simulink model "swirling_pendulum_PFL_acrobot_spong_based_collocated"  (R2021a)
settings: Solver=ode2  StartTime=0.0  StopTime=40  FixedStep=1e-4  RelTol=1e-3
undefined symbols (not defined in the file or in its folder): sigbuilder_block, X, Y, Z
libraries: sm_lib x15, nesl_utility x3, dspswit3 x1
settings Model: Creator=aarti  LastModifiedBy=Riswadkar
settings SolverCC: ZeroCrossControl=DisableAll
settings DataIOCC: SaveState=on  ReturnWorkspaceOutputs=off

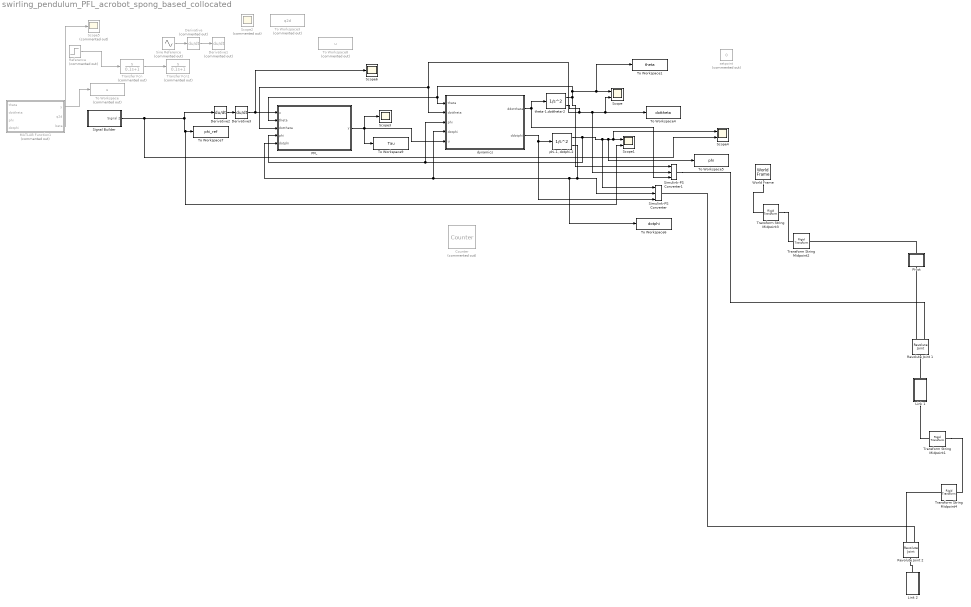
== system swirling_pendulum_PFL_acrobot_spong_based_collocated ==
  Counter : dspswit3/Counter  Commented=on  Direction=Up  CountEvent=Rising edge  CounterSize=User defined  MaxCount=255  InitialCount=0  Output=Count and Hit  HitValue=32  ResetInput=on  SamplesPerFrame=1  Ts=1  CntDtype=double  HitDtype=Logical
  Derivative : Derivative  Commented=on
  Derivative1 : Derivative  Commented=on
  Derivative2 : Derivative
  Derivative3 : Derivative
  Link 1 : Subsystem  Tag=CustomStyle
  Link 2 : Subsystem  Tag=CustomStyle
  MATLAB Function1 : MATLAB Function  Commented=on  TreatAsAtomicUnit=on
  PFL : MATLAB Function  TreatAsAtomicUnit=on
  Pivot : Subsystem  Tag=CustomStyle
  Reference : Step  Commented=on  Time=2  After=pi/2  SampleTime=0
  Revolute Joint 1 : sm_lib/Joints/Revolute Joint  JointMode=Normal  SenseConstraintForce=off  SenseConstraintForceX=off  SenseConstraintForceY=off  SenseConstraintForceZ=off  SenseConstraintTorque=off  SenseConstraintTorqueX=off  SenseConstraintTorqueY=off  SenseConstraintTorqueZ=off  SenseTotalForce=off  SenseTotalForceX=off  SenseTotalForceY=off  SenseTotalForceZ=off  SenseTotalTorque=off  SenseTotalTorqueX=off  SenseTotalTorqueY=off  SenseTotalTorqueZ=off  CompositeWrenchDir=FollowerOnBase  CompositeWrenchFrame=BaseFrame  EquilibriumPosition=0  EquilibriumPositionUnits=rad  SpringStiffness=0  SpringStiffnessUnits=N*m/rad  DampingCoefficient=0  DampingCoefficientUnits=N*m/(rad/s)  TorqueActuationMode=ComputedTorque  MotionActuationMode=InputMotion  SensePosition=off  SenseVelocity=off  SenseAcceleration=off  SenseTorqueForce=off  SenseLowerLimitTorqueForce=off  SenseUpperLimitTorqueForce=off  LowerLimitSpecify=off  LowerLimitBound=-90  LowerLimitBoundUnits=deg  LowerLimitStiffness=1e4  LowerLimitStiffnessUnits=N*m/deg  LowerLimitDamping=10  LowerLimitDampingUnits=N*m/(deg/s)  LowerLimitTransitionRegionWidth=0.1  LowerLimitTransitionRegionWidthUnits=deg  UpperLimitSpecify=off  UpperLimitBound=90  UpperLimitBoundUnits=deg  UpperLimitStiffness=1e4  UpperLimitStiffnessUnits=N*m/deg  UpperLimitDamping=10  UpperLimitDampingUnits=N*m/(deg/s)  UpperLimitTransitionRegionWidth=0.1  UpperLimitTransitionRegionWidthUnits=deg  PositionTargetSpecify=off  PositionTargetPriority=High  PositionTargetValue=0  PositionTargetValueUnits=deg  VelocityTargetSpecify=off  VelocityTargetPriority=High  VelocityTargetValue=0  VelocityTargetValueUnits=rad/s
  Revolute Joint 2 : sm_lib/Joints/Revolute Joint  JointMode=Normal  SenseConstraintForce=off  SenseConstraintForceX=off  SenseConstraintForceY=off  SenseConstraintForceZ=off  SenseConstraintTorque=off  SenseConstraintTorqueX=off  SenseConstraintTorqueY=off  SenseConstraintTorqueZ=off  SenseTotalForce=off  SenseTotalForceX=off  SenseTotalForceY=off  SenseTotalForceZ=off  SenseTotalTorque=off  SenseTotalTorqueX=off  SenseTotalTorqueY=off  SenseTotalTorqueZ=off  CompositeWrenchDir=FollowerOnBase  CompositeWrenchFrame=BaseFrame  EquilibriumPosition=0  EquilibriumPositionUnits=rad  SpringStiffness=0  SpringStiffnessUnits=N*m/rad  DampingCoefficient=0  DampingCoefficientUnits=N*m/(rad/s)  TorqueActuationMode=ComputedTorque  MotionActuationMode=InputMotion  SensePosition=off  SenseVelocity=off  SenseAcceleration=off  SenseTorqueForce=off  SenseLowerLimitTorqueForce=off  SenseUpperLimitTorqueForce=off  LowerLimitSpecify=off  LowerLimitBound=-90  LowerLimitBoundUnits=deg  LowerLimitStiffness=1e4  LowerLimitStiffnessUnits=N*m/deg  LowerLimitDamping=10  LowerLimitDampingUnits=N*m/(deg/s)  LowerLimitTransitionRegionWidth=0.1  LowerLimitTransitionRegionWidthUnits=deg  UpperLimitSpecify=off  UpperLimitBound=90  UpperLimitBoundUnits=deg  UpperLimitStiffness=1e4  UpperLimitStiffnessUnits=N*m/deg  UpperLimitDamping=10  UpperLimitDampingUnits=N*m/(deg/s)  UpperLimitTransitionRegionWidth=0.1  UpperLimitTransitionRegionWidthUnits=deg  PositionTargetSpecify=off  PositionTargetPriority=High  PositionTargetValue=0  PositionTargetValueUnits=deg  VelocityTargetSpecify=off  VelocityTargetPriority=High  VelocityTargetValue=0  VelocityTargetValueUnits=rad/s
  Scope : Scope  NumInputPorts=2
  Scope1 : Scope  NumInputPorts=2
  Scope2 : Scope  Commented=on
  Scope3 : Scope
  Scope4 : Scope  NumInputPorts=2
  Scope5 : Scope  Commented=on
  Scope6 : Scope
  Signal Builder : Subsystem  Tag=STV Subsys  LoadFcn=sigbuilder_block('load');  StartFcn=sigbuilder_block('start');  StopFcn=sigbuilder_block('stop');  ClipboardFcn=sigbuilder_block('clipboard');  mask(Sigbuilder block){tuvar=[0:10]}
      mask help: Simulink:masks:SigbuilderBlock_MD
      mask init:
      | if ~strcmp(get_param(bdroot(gcbh),'SimulationStatus'),'stopped') tuvar = sigbuilder_block('maskInit'); end
      settings: CopyFcn=sigbuilder_block('copy');  DeleteFcn=sigbuilder_block('delete');  ModelCloseFcn=sigbuilder_block('modelClose');  PreSaveFcn=sigbuilder_block('preSave');  PauseFcn=sigbuilder_block('pause');  ContinueFcn=sigbuilder_block('continue');  NameChangeFcn=sigbuilder_block('namechange');  OpenFcn=sigbuilder_block('open',[5.4 36 1141.2 516.6 ]);  CloseFcn=sigbuilder_block('close');
      mask Display: plot(0, 0, 100, 100,[2, 2, 32, 32, 2], [68, 8, 8, 68, 68],[32, 2], [38, 38], [32, 19, 2],[53, 60, 44], [32, 17, 17, 2],[16, 16, 31, 31]);txt = getActiveGroup(gcbh);text(2, 100, txt,'verticalAlignment', 'top');
  Simulink-PS Converter : nesl_utility/Simulink-PS Converter  PhysicalDomain=network_engine_domain  SubClassName=ps_input  LeftPortType=input  RightPortType=output  PseudoPeriodic=off  Frequencies=[]  NoiseDistribution=none  NoiseParameters=[]  Unit=1  AffineConversion=off  FilteringAndDerivatives=provide  SimscapeFilterOrder=1  InputFilterTimeConstant=0.001  UdotUserProvided=2
      settings: SourceProductBaseCode=PW,SS
  Simulink-PS Converter1 : nesl_utility/Simulink-PS Converter  PhysicalDomain=network_engine_domain  SubClassName=ps_input  LeftPortType=input  RightPortType=output  PseudoPeriodic=off  Frequencies=[]  NoiseDistribution=none  NoiseParameters=[]  Unit=1  AffineConversion=off  FilteringAndDerivatives=provide  SimscapeFilterOrder=1  InputFilterTimeConstant=0.001  UdotUserProvided=2
      settings: SourceProductBaseCode=PW,SS
  Sine Reference : Sin  Commented=on  SampleTime=0
  To Workspace : ToWorkspace  Commented=on  VariableName=u  SampleTime=-1
  To Workspace1 : ToWorkspace  VariableName=theta  SampleTime=-1
  To Workspace3 : ToWorkspace  Commented=on  VariableName=q2d  SampleTime=-1
  To Workspace4 : ToWorkspace  VariableName=dottheta  SampleTime=-1
  To Workspace5 : ToWorkspace  VariableName=phi  SampleTime=-1
  To Workspace6 : ToWorkspace  VariableName=dotphi  SampleTime=-1
  To Workspace7 : ToWorkspace  VariableName=phi_ref  SampleTime=-1
  To Workspace8 : ToWorkspace  Commented=on  VariableName=u  SampleTime=-1
  To Workspace9 : ToWorkspace  VariableName=Tau  SampleTime=-1
  Transfer Fcn : TransferFcn  Commented=on  Numerator=[1 0]  Denominator=[0.1 1]
  Transfer Fcn1 : TransferFcn  Commented=on  Numerator=[1 0]  Denominator=[0.1 1]
  Transform String Midpoint1 : sm_lib/Frames and Transforms/Rigid Transform  TranslationMethod=None  TranslationStandardOffset=0  TranslationLengthUnit=m  TranslationStandardAxis=-Y  TranslationCartesianOffset=[0 0 0]  TranslationROffset=0  TranslationROffsetUnits=m  TranslationZOffset=0  TranslationZOffsetUnits=m  TranslationThetaOffset=0  TranslationThetaOffsetUnits=deg  RotationMethod=StandardAxis  RotationAngleUnits=deg  RotationStandardAxis=-X  RotationAngle=90  RotationArbitraryAxis=[0 0 1]  FollAlignAxisA=+X  BaseAlignAxisA=+Y  FollAlignAxisB=+Y  BaseAlignAxisB=+Z  RotationSequenceAxes=FollowerAxes  RotationSequence=XYX  RotationSequenceAngles=[0 0 0]  RotationSequenceAnglesUnits=deg  RotationMatrix=[1 0 0; 0 1 0; 0 0 1]
  Transform String Midpoint2 : sm_lib/Frames and Transforms/Rigid Transform  TranslationMethod=None  TranslationStandardOffset=0  TranslationLengthUnit=m  TranslationStandardAxis=-Y  TranslationCartesianOffset=[0 0 0]  TranslationROffset=0  TranslationROffsetUnits=m  TranslationZOffset=0  TranslationZOffsetUnits=m  TranslationThetaOffset=0  TranslationThetaOffsetUnits=deg  RotationMethod=StandardAxis  RotationAngleUnits=deg  RotationStandardAxis=+X  RotationAngle=90  RotationArbitraryAxis=[0 0 1]  FollAlignAxisA=+X  BaseAlignAxisA=+Y  FollAlignAxisB=+Y  BaseAlignAxisB=+Z  RotationSequenceAxes=FollowerAxes  RotationSequence=XYX  RotationSequenceAngles=[0 0 0]  RotationSequenceAnglesUnits=deg  RotationMatrix=[1 0 0; 0 1 0; 0 0 1]
  Transform String Midpoint3 : sm_lib/Frames and Transforms/Rigid Transform  TranslationMethod=None  TranslationStandardOffset=0  TranslationLengthUnit=m  TranslationStandardAxis=-Y  TranslationCartesianOffset=[0 0 0]  TranslationROffset=0  TranslationROffsetUnits=m  TranslationZOffset=0  TranslationZOffsetUnits=m  TranslationThetaOffset=0  TranslationThetaOffsetUnits=deg  RotationMethod=StandardAxis  RotationAngleUnits=deg  RotationStandardAxis=+Y  RotationAngle=180  RotationArbitraryAxis=[0 0 1]  FollAlignAxisA=+X  BaseAlignAxisA=+Y  FollAlignAxisB=+Y  BaseAlignAxisB=+Z  RotationSequenceAxes=FollowerAxes  RotationSequence=XYX  RotationSequenceAngles=[0 0 0]  RotationSequenceAnglesUnits=deg  RotationMatrix=[1 0 0; 0 1 0; 0 0 1]
  Transform String Midpoint4 : sm_lib/Frames and Transforms/Rigid Transform  TranslationMethod=None  TranslationStandardOffset=0.15/2  TranslationLengthUnit=m  TranslationStandardAxis=-Y  TranslationCartesianOffset=[0 0 0]  TranslationROffset=0  TranslationROffsetUnits=m  TranslationZOffset=0  TranslationZOffsetUnits=m  TranslationThetaOffset=0  TranslationThetaOffsetUnits=deg  RotationMethod=StandardAxis  RotationAngleUnits=deg  RotationStandardAxis=-X  RotationAngle=180  RotationArbitraryAxis=[0 0 1]  FollAlignAxisA=+X  BaseAlignAxisA=+Y  FollAlignAxisB=+Y  BaseAlignAxisB=+Z  RotationSequenceAxes=FollowerAxes  RotationSequence=XYX  RotationSequenceAngles=[0 0 0]  RotationSequenceAnglesUnits=deg  RotationMatrix=[1 0 0; 0 1 0; 0 0 1]
  World Frame : sm_lib/Frames and Transforms/World Frame
  dynamics : MATLAB Function  TreatAsAtomicUnit=on
  "phi-1, dotphi-2" : SecondOrderIntegrator  ICX=0  WrapX=on  ICDXDT=0
  setpoint : Constant  Commented=on  Value=0
  theta-1,dottheta-2 : SecondOrderIntegrator  ICX=0  WrapX=on  ICDXDT=0
  wires:
  dynamics/1(ddottheta) -> Simulink-PS Converter1/3, theta-1,dottheta-2/1
  dynamics/2(ddotphi) -> Simulink-PS Converter/3, "phi-1, dotphi-2"/1
  theta-1,dottheta-2/2 -> PFL/3(dottheta), dynamics/2(dottheta), Simulink-PS Converter1/2, To Workspace4/1, Scope/2
  "phi-1, dotphi-2"/1 -> Simulink-PS Converter/1, To Workspace5/1, Scope4/1, Scope1/1, dynamics/3(phi), PFL/4(phi)
  "phi-1, dotphi-2"/2 -> To Workspace6/1, dynamics/4(dotphi), PFL/5(dotphi), Simulink-PS Converter/2
  theta-1,dottheta-2/1 -> Simulink-PS Converter1/1, To Workspace1/1, Scope/1, PFL/2(theta), dynamics/1(theta)
  PFL/1(y) -> To Workspace9/1, Scope3/1, dynamics/5(u)
  Reference/1 -> Transfer Fcn/1
  Transfer Fcn/1 -> Transfer Fcn1/1
  Sine Reference/1 -> Derivative/1
  Derivative/1 -> Derivative1/1
  Derivative2/1 -> Derivative3/1
  MATLAB Function1/1(y) -> To Workspace/1
  MATLAB Function1/3(beta) -> Scope5/1
  Derivative3/1 -> Scope6/1, PFL/1(u)
  Signal Builder/1(Signal 2) -> Scope4/2, Derivative2/1, Scope1/2, To Workspace7/1
  connections:
  Pivot/RConn1 -- Revolute Joint 1/LConn1
  Link 2/RConn1 -- Revolute Joint 2/RConn1
  World Frame/RConn1 -- Transform String Midpoint3/RConn1
  Simulink-PS Converter1/RConn1 -- Revolute Joint 1/LConn2
  Link 1/RConn1 -- Revolute Joint 1/RConn1
  Transform String Midpoint1/LConn1 -- Transform String Midpoint4/LConn1
  Link 1/LConn1 -- Transform String Midpoint1/RConn1
  Revolute Joint 2/LConn2 -- Simulink-PS Converter/RConn1
  Transform String Midpoint3/LConn1 -- Transform String Midpoint2/RConn1
  Pivot/LConn1 -- Transform String Midpoint2/LConn1
  Transform String Midpoint4/RConn1 -- Revolute Joint 2/LConn1

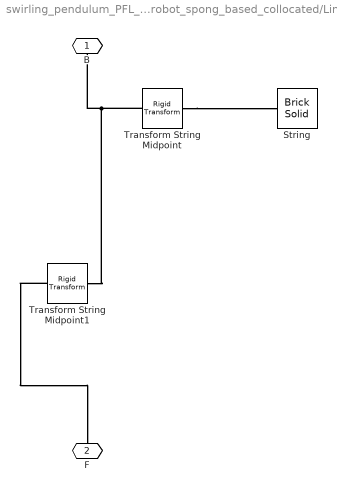
== system swirling_pendulum_PFL_acrobot_spong_based_collocated/Link 1 ==
  String : sm_lib/Body Elements/Brick Solid  GraphicAmbientColor=[0.15 0.15 0.15 1.0]  BasedOnType=Density  BrickDimensions=[0.012 0.25 0.012]  BrickDimensionUnits=m  CenterOfMass=[0 0 0]  CenterOfMassUnits=m  GraphicDiffuseColor=[0.3764706 0.21568628 0.3764706]  Density=0  DensityUnits=kg/(m^3)  DoExposeReferenceFrame=on  GraphicEmissiveColor=[0.0 0.0 0.0 1.0]  ExportEntireGeometry=off  SerializedFrames=<Frames/>  MarkerShape=Sphere  MarkerSize=10  GraphicType=FromGeometry  InertiaType=PointMass  Mass=0  MassUnits=kg  MomentsOfInertia=[1 1 1]*1e-3  MomentsOfInertiaUnits=kg*m^2  GraphicOpacity=1.0  ProductsOfInertia=[0 0 0]  ProductsOfInertiaUnits=kg*m^2  GraphicShininess=75  GraphicSpecularColor=[0.5 0.5 0.5 1.0]  GraphicVisPropType=SimpleVisualProperties
  Transform String Midpoint : sm_lib/Frames and Transforms/Rigid Transform  TranslationMethod=StandardAxis  TranslationStandardOffset=0.25/2  TranslationLengthUnit=m  TranslationStandardAxis=-Y  TranslationCartesianOffset=[0 0 0]  TranslationROffset=0  TranslationROffsetUnits=m  TranslationZOffset=0  TranslationZOffsetUnits=m  TranslationThetaOffset=0  TranslationThetaOffsetUnits=deg  RotationMethod=None  RotationAngleUnits=deg  RotationStandardAxis=+Z  RotationAngle=0  RotationArbitraryAxis=[0 0 1]  FollAlignAxisA=+X  BaseAlignAxisA=+Y  FollAlignAxisB=+Y  BaseAlignAxisB=+Z  RotationSequenceAxes=FollowerAxes  RotationSequence=XYX  RotationSequenceAngles=[0 0 0]  RotationSequenceAnglesUnits=deg  RotationMatrix=[1 0 0; 0 1 0; 0 0 1]
  Transform String Midpoint1 : sm_lib/Frames and Transforms/Rigid Transform  TranslationMethod=StandardAxis  TranslationStandardOffset=0.25  TranslationLengthUnit=m  TranslationStandardAxis=-Y  TranslationCartesianOffset=[0 0 0]  TranslationROffset=0  TranslationROffsetUnits=m  TranslationZOffset=0  TranslationZOffsetUnits=m  TranslationThetaOffset=0  TranslationThetaOffsetUnits=deg  RotationMethod=None  RotationAngleUnits=deg  RotationStandardAxis=+Z  RotationAngle=0  RotationArbitraryAxis=[0 0 1]  FollAlignAxisA=+X  BaseAlignAxisA=+Y  FollAlignAxisB=+Y  BaseAlignAxisB=+Z  RotationSequenceAxes=FollowerAxes  RotationSequence=XYX  RotationSequenceAngles=[0 0 0]  RotationSequenceAnglesUnits=deg  RotationMatrix=[1 0 0; 0 1 0; 0 0 1]
  B : PMIOPort  Side=Right
  F : PMIOPort  Port=2  Side=Left
  connections:
  Transform String Midpoint/RConn1 -- String/RConn1
  Transform String Midpoint/LConn1 -- Transform String Midpoint1/LConn1 -- B/RConn1
  Transform String Midpoint1/RConn1 -- F/RConn1

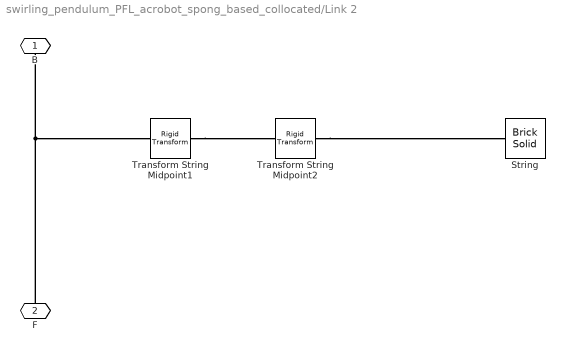
== system swirling_pendulum_PFL_acrobot_spong_based_collocated/Link 2 ==
  String : sm_lib/Body Elements/Brick Solid  GraphicAmbientColor=[0.15 0.15 0.15 1.0]  BasedOnType=Density  BrickDimensions=[0.015 0.15 0.015]  BrickDimensionUnits=m  CenterOfMass=[0 0 0]  CenterOfMassUnits=m  GraphicDiffuseColor=[0.011764706 0.40392157 0.6392157]  Density=0  DensityUnits=kg/(m^3)  DoExposeReferenceFrame=on  GraphicEmissiveColor=[0.0 0.0 0.0 1.0]  ExportEntireGeometry=off  SerializedFrames=<Frames/>  MarkerShape=Sphere  MarkerSize=10  GraphicType=FromGeometry  InertiaType=PointMass  Mass=0  MassUnits=kg  MomentsOfInertia=[1 1 1]*1e-3  MomentsOfInertiaUnits=kg*m^2  GraphicOpacity=1.0  ProductsOfInertia=[0 0 0]  ProductsOfInertiaUnits=kg*m^2  GraphicShininess=75  GraphicSpecularColor=[0.5 0.5 0.5 1.0]  GraphicVisPropType=SimpleVisualProperties
  Transform String Midpoint1 : sm_lib/Frames and Transforms/Rigid Transform  TranslationMethod=StandardAxis  TranslationStandardOffset=0.15/2  TranslationLengthUnit=m  TranslationStandardAxis=-Y  TranslationCartesianOffset=[0 0 0]  TranslationROffset=0  TranslationROffsetUnits=m  TranslationZOffset=0  TranslationZOffsetUnits=m  TranslationThetaOffset=0  TranslationThetaOffsetUnits=deg  RotationMethod=StandardAxis  RotationAngleUnits=deg  RotationStandardAxis=-Z  RotationAngle=180  RotationArbitraryAxis=[0 0 1]  FollAlignAxisA=+X  BaseAlignAxisA=+Y  FollAlignAxisB=+Y  BaseAlignAxisB=+Z  RotationSequenceAxes=FollowerAxes  RotationSequence=XYX  RotationSequenceAngles=[0 0 0]  RotationSequenceAnglesUnits=deg  RotationMatrix=[1 0 0; 0 1 0; 0 0 1]
  Transform String Midpoint2 : sm_lib/Frames and Transforms/Rigid Transform  TranslationMethod=None  TranslationStandardOffset=0.15/2  TranslationLengthUnit=m  TranslationStandardAxis=-Y  TranslationCartesianOffset=[0 0 0]  TranslationROffset=0  TranslationROffsetUnits=m  TranslationZOffset=0  TranslationZOffsetUnits=m  TranslationThetaOffset=0  TranslationThetaOffsetUnits=deg  RotationMethod=StandardAxis  RotationAngleUnits=deg  RotationStandardAxis=+X  RotationAngle=0  RotationArbitraryAxis=[0 0 1]  FollAlignAxisA=+X  BaseAlignAxisA=+Y  FollAlignAxisB=+Y  BaseAlignAxisB=+Z  RotationSequenceAxes=FollowerAxes  RotationSequence=XYX  RotationSequenceAngles=[0 0 0]  RotationSequenceAnglesUnits=deg  RotationMatrix=[1 0 0; 0 1 0; 0 0 1]
  B : PMIOPort  Side=Right
  F : PMIOPort  Port=2  Side=Left
  connections:
  Transform String Midpoint1/LConn1 -- Transform String Midpoint2/RConn1
  F/RConn1 -- Transform String Midpoint1/RConn1 -- B/RConn1
  Transform String Midpoint2/LConn1 -- String/RConn1

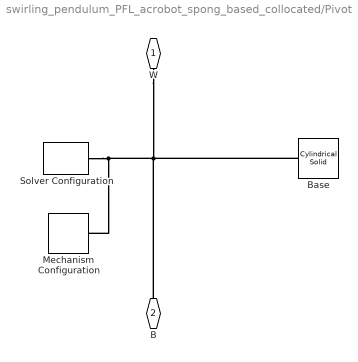
== system swirling_pendulum_PFL_acrobot_spong_based_collocated/Pivot ==
  Base : sm_lib/Body Elements/Cylindrical Solid  GraphicAmbientColor=[0.15 0.15 0.15 1.0]  BasedOnType=Density  CenterOfMass=[0 0 0]  CenterOfMassUnits=m  GraphicDiffuseColor=[0.3 0.3 0.3]  CylinderLength=0.4  CylinderLengthUnits=m  CylinderRadius=0.01  CylinderRadiusUnits=m  Density=1000  DensityUnits=kg/(m^3)  DoExposeReferenceFrame=on  GraphicEmissiveColor=[0.0 0.0 0.0 1.0]  ExportEntireGeometry=off  SerializedFrames=<Frames/>  MarkerShape=Sphere  MarkerSize=10  GraphicType=FromGeometry  InertiaType=PointMass  Mass=10  MassUnits=kg  MomentsOfInertia=[1 1 1]*1e-3  MomentsOfInertiaUnits=kg*m^2  GraphicOpacity=1.0  ProductsOfInertia=[0 0 0]  ProductsOfInertiaUnits=kg*m^2  GraphicShininess=75  GraphicSpecularColor=[0.5 0.5 0.5 1.0]  GraphicVisPropType=AdvancedVisualProperties
  Mechanism Configuration : sm_lib/Utilities/Mechanism Configuration  UniformGravity=Constant  GravityVector=[0 0 -9.81]  GravityVectorUnits=m/s^2  GravityUnits=m/s^2  LinearizationDelta=0.001  JointModeTransitionNonlinearIterations=2
  Solver Configuration : nesl_utility/Solver Configuration  PhysicalDomain=network_engine_domain  SubClassName=solver  LeftPortType=input  RightPortType=generic  Tones=[]  Harmonics=[]  SimulateNoise=off  Profile=off  UseLocalSampling=off  EnableSwitchedLinearOptims=on  FrequencyDomain=off  UseCCode=off  RelTol=0.001  AbsTol=1e-06  MinStep=1e-09  ToWorkspace=off  RevertToSquareIcSolve=off  NumHomotopyIterations=100  PhasorMode=off  PhasorModeNumHarmonics=1  DoDC=on  ResidualTolerance=1e-9  UseLocalSolver=off  LocalSolverChoice=NE_BACKWARD_EULER_ADVANCER  LocalSolverSampleTime=.001  DoFixedCost=off  MaxNonlinIter=3  MaxModeIter=2  ComputeImpulses=off  ImpulseIterations=2  LinearAlgebra=Sparse  EquationFormulation=NE_TIME_EF  DelaysMemoryBudget=1024  AutomaticFiltering=on  FilteringTimeConstant=0.001  PartitionStorageMethod=AS_NEEDED  PartitionMemoryBudget=1024  PartitionMethod=FAST
      settings: SourceProductBaseCode=PW,SS
  W : PMIOPort  Side=Left
  B : PMIOPort  Port=2  Side=Right
  connections:
  W/RConn1 -- B/RConn1 -- Base/RConn1 -- Solver Configuration/RConn1 -- Mechanism Configuration/RConn1

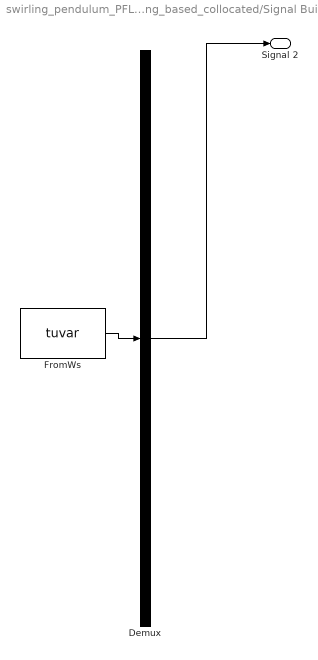
== system swirling_pendulum_PFL_acrobot_spong_based_collocated/Signal Builder ==
  Demux : Demux  Tag=STV Demux  Outputs=1
      settings: DisplayOption=none
  FromWs : FromWorkspace  Tag=STV FromWs  VariableName=tuvar
      SigBuilderData=|
      | common.afterFinalStr = 'Extrapolate'
      | common.sampleTime = 0
      | dataSet.timeRange = [0 40]
      | dataSet.name = 'Group 1'
      | sbobj.Groups.Name = 'Group 1'
      | sbobj.Groups.Signals.Name = 'Signal 2'
      | sbobj.Groups.Signals.XData = [0 0.01 0.02 0.03 0.04 0.05 0.06 0.07 0.08 0.09 0.1 0.11 ... (3002 elements, 1x3002)]
      | sbobj.Groups.Signals.YData = [0 0.0314107590781 0.0627905195293 0.0941083133185 0.125333233564 0.15643446504 0.187381314586 0.218143241397 0.248689887165 0.278991106039 0.309016994375 0.338737920245 ... (3002 elements, 1x3002)]
      | sbobj.Groups.TimeRange = [0 40]
  Signal 2 : Outport  Tag=STV Outport
  wires:
  FromWs/1 -> Demux/1
  Demux/1 -> Signal 2/1

== matlab function swirling_pendulum_PFL_acrobot_spong_based_collocated/dynamics ==
  data: theta input; ddottheta output; dottheta input; phi input; dotphi input; u input; ddotphi output
function [ddottheta,ddotphi]=SwirlingPendulum(theta,dottheta,phi,dotphi,u)
%% Swirling Pendulum Equations of Motion
%Define the parameter values
% m1 = 0.435;
% m2 = 0.325;
% l1 = 0.07;
% l2 = 0.0855 ;
% g = 9.81;
m1 = 0.01353; 
m2 = 0.209; 
l1 =0.093; 
l2 =0.114;
% b1 = 0.002 ;
% b2 = 0.002 ;
g = 9.81; 
% Inertia Matrix
    M=[4/3*(m1*l1^2+m2*(3*l1^2+(l2*sin(phi))^2)), 2*m2*l1*l2*cos(phi);
    2*m2*l1*l2*cos(phi), 4/3*(m2*l2^2)];
% Coriolis 
    C = [(4/3)*m2*l2*l2*sin(phi)*cos(phi)*dotphi, (4/3)*m2*l2*l2*sin(phi)*cos(phi)*dottheta - 2*m2*l1*l2*sin(phi)*dotphi;
    (-4/3)*m2*l2*l2*cos(phi)*sin(phi)*dottheta, 0];
% Potential Terms
    G=[(m1+2*m2)*g*l1*sin(theta)+m2*g*l2*sin(phi)*cos(theta);m2*g*l2*sin(theta)*cos(phi)];
% % Viscous friction
%     D = [b1*dottheta;b2*dotphi] ;
%Mx''+Cx'+G+D = Bu;
B = [0;1] ;
ddotX=inv(M)*(-C*[dottheta;dotphi]-G+B*u);
ddottheta=ddotX(1,:);
ddotphi=ddotX(2,:);

== matlab function swirling_pendulum_PFL_acrobot_spong_based_collocated/PFL ==
  data: u input; y output; theta input; dottheta input; phi input; dotphi input
function y = fcn(u,theta,dottheta,phi,dotphi)
% m1 = 0.435;
% m2 = 0.325;
% l1 = 0.07;
% l2 = 0.0855 ;
% g = 9.81;
m1 = 0.01353 ; 
m2 = 0.209 ; 
l1 =0.093 ; 
l2 =0.114 ; 
g = 9.81 ;
% b1 = 0.002 ;
% b2 = 0.002 ;
% Inertia Matrix
    M=[4/3*(m1*l1^2+m2*(3*l1^2+(l2*sin(phi))^2)), 2*m2*l1*l2*cos(phi);
    2*m2*l1*l2*cos(phi), 4/3*(m2*l2^2)];
% Coriolis 
    C = [(4/3)*m2*l2*l2*sin(phi)*cos(phi)*dotphi, (4/3)*m2*l2*l2*sin(phi)*cos(phi)*dottheta - 2*m2*l1*l2*sin(phi)*dotphi;
    (-4/3)*m2*l2*l2*cos(phi)*sin(phi)*dottheta, 0];
% Potential Terms
    G=[(m1+2*m2)*g*l1*sin(theta)+m2*g*l2*sin(phi)*cos(theta);m2*g*l2*sin(theta)*cos(phi)];
d22_p = M(2,2) - (M(2,1)*M(1,2))/M(1,1) ;
h1 = C(1,1)*dottheta + C(1,2)*dotphi ;
h2 = C(2,1)*dottheta + C(2,2)*dotphi ;
c2_p = h2 - (M(2,1)*h1)/M(1,1) ;
g2_p = G(2,1) - (M(2,1)*G(1,1))/M(1,1) ;
% b2_p = b2*dotphi - (M(2,1)*b1*dottheta)/M(1,1) ;
Tau = d22_p*u + c2_p + g2_p  ;
y = Tau ;
end

== matlab function swirling_pendulum_PFL_acrobot_spong_based_collocated/MATLAB Function1 ==
  data: theta input; y output; q2d output; dottheta input; phi input; dotphi input; beta output
function [y,q2d,beta] = fcn(theta,dottheta,phi,dotphi)
% previoustheta = 0 ;
% currenttheta = theta ;
% inc = 0;
% if((currenttheta - previoustheta) > pi/180 )
%     inc = 1 ;
% end
% previoustheta = currenttheta ;
flag = 0 ;
Ed = 0.7451 ;
K = 10 ;
m1 = 0.01353; m2 = 0.209; l1 =0.093; l2 =0.114; g = 9.81;
flag1 = 0 ;
%% For wrapping of theta and phi between [0,2*pi]
beta = mod(theta, 2*pi) ;
gamma = mod(phi, 2*pi) ;
%% Swing-up control 
Kp = 85 ;
Kd = 10 ;
% Kp = 200 ;
% Kd = 200 ;
alpha = pi ;  % desired value of theta
q2d = 2*(alpha/pi)*atan(dottheta) ; % setpoint for link 2
% q2d = pi/4 ;
% q2d = pi ;
if((flag == 0)&&(flag1 == 0))
    y = Kp*(q2d - phi) - Kd*dotphi; % swing-up controller feedback based
end
E = (m1+2*m2)*g*l1*cos(theta) + m2*g*l2*sin(phi)*sin(theta);

%% Stabilizing controller
if(((abs(beta) > 5 * pi/6 ) && (abs(beta) < pi))||(flag == 1))
    flag = 1 ;
    if(((abs(beta) > pi)&&(abs(beta) < 2*pi))&&(E > Ed))
        y = - K*dottheta*(E - Ed) ;
    end    
    x = [beta-pi;phi-0;dottheta-0;dotphi-0] ;
    K1 = [-8.4449   -2.7530   -0.3457    0.9407] ;
    y = - K1*x ;
end
end
